simulink subsystem "Laseres"  (R2023b)
settings: Solver=VariableStepAuto  StartTime=0.0  StopTime=10.0  RelTol=1e-3
settings Model: Creator=migue  LastModifiedBy=Andrés

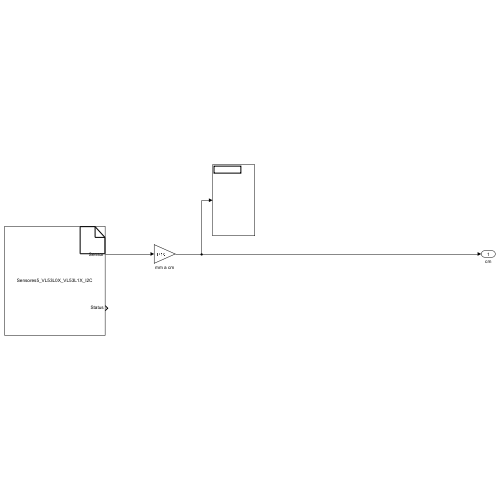
[thumbnail: Simulink's stored preview of the top-level diagram]
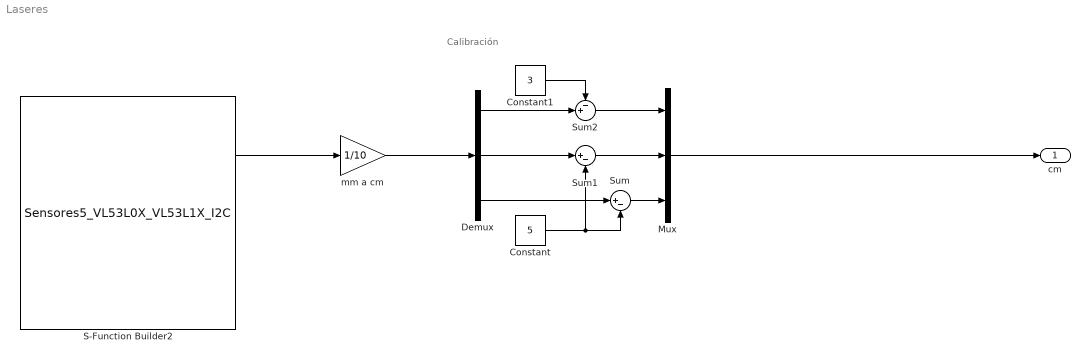
== system Laseres ==
  note: Calibración
  Constant : Constant  Value=5
  Constant1 : Constant  Value=3
  Demux : Demux  Outputs=3
  Mux : Mux  Inputs=3
  S-Function Builder2 : S-Function  InitFcn=try, set_param(gcb,'FunctionName','Sensores5_VL53L0X_VL53L1X_I2C'), end  FunctionName=Sensores5_VL53L0X_VL53L1X_I2C  SFunctionModules=Sensores5_VL53L0X_VL53L1X_I2C_wrapper.cpp  SFunctionDeploymentMode=off  EnableBusSupport=off  mask(S-Function Builder){}
      mask help: Simulink:masks:SFunctionBuilder_MD
      mask init:
      | val = [[.9  0.75 0.75 1 1 .9 .9 1]',[1 1 0.75 0.75 .9 .9 1 .9]'];try , sys = get_param(gcb,'SfunBuilderFcnName');if isempty(sys), sys = get_param(gcb,'FunctionName'); end,catch, sys = get_param(gcb,'FunctionName'); end
      settings: CopyFcn=set_param(gcbh,'LinkStatus','none')  PreSaveFcn=try, set_param(gcb,'FunctionName','Sensores5_VL53L0X_VL53L1X_I2C'), end  OpenFcn=sfunctionwizard(gcbh)
      mask Display:
      | plot(val(:,1),val(:,2))
      | disp(sys)
      | port_label('output',1,'Sensor')
      | port_label('output',2,'Status')
  Sum : Sum  Inputs=|+-
  Sum1 : Sum  Inputs=|+-
  Sum2 : Sum  Inputs=-+|
  mm a cm : Gain  Gain=1/10
  cm : Outport
  wires:
  S-Function Builder2/1 -> mm a cm/1
  mm a cm/1 -> Demux/1
  Demux/3 -> Sum/1
  Constant/1 -> Sum1/2, Sum/2
  Demux/2 -> Sum1/1
  Sum1/1 -> Mux/2
  Sum/1 -> Mux/3
  Demux/1 -> Sum2/2
  Sum2/1 -> Mux/1
  Constant1/1 -> Sum2/1
  Mux/1 -> cm/1
